simulink model "Tarea1-Simulacion"  (R2021b)
settings: Solver=VariableStepAuto  StartTime=0.0  StopTime=10  RelTol=1e-3
values from neighbouring files (symbols this model uses):
  Kc = Ksc (1:2)    [Tarea1-Marco_Rodriguez.m]
  Kd = Ksd (1:2)    [Tarea1-Marco_Rodriguez.m]
undefined symbols (not defined in the file or in its folder): DiscIntNeverNeededParam
libraries: cstblocks x10
settings Model: Creator=mvrb9  LastModifiedBy=mvrb9

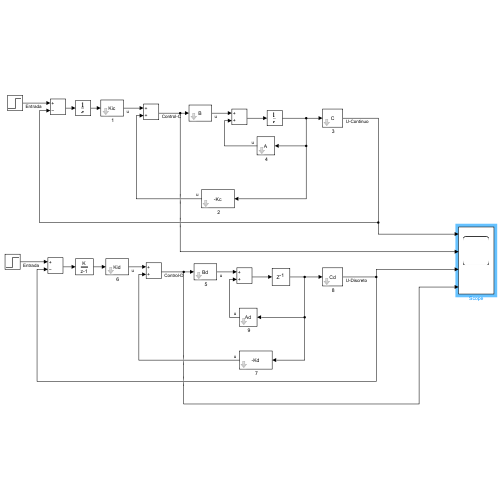
[thumbnail: Simulink's stored preview of the top-level diagram]
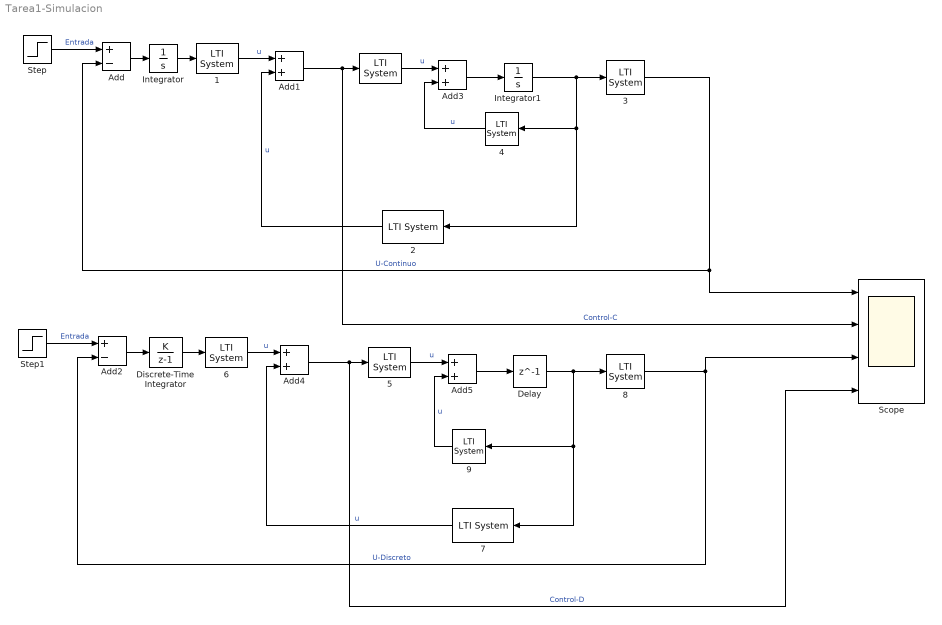
== system Tarea1-Simulacion ==
  " " : cstblocks/LTI System  sys=B  IC=[]
  " 1" : cstblocks/LTI System  sys=Kic  IC=[]
  " 2" : cstblocks/LTI System  sys=-Kc  IC=[]
  " 3" : cstblocks/LTI System  sys=C  IC=[]
  " 4" : cstblocks/LTI System  sys=A  IC=[]
  " 5" : cstblocks/LTI System  sys=Bd  IC=[]
  " 6" : cstblocks/LTI System  sys=Kid  IC=[]
  " 7" : cstblocks/LTI System  sys=-Kd  IC=[]
  " 8" : cstblocks/LTI System  sys=Cd  IC=[]
  " 9" : cstblocks/LTI System  sys=Ad  IC=[]
  Add : Sum  Inputs=+-
  Add{1,3..5} (4 alike) : Sum
  Add2 : Sum  Inputs=+-
  Delay : Delay  DelayLength=1  InitialCondition=0  SampleTime=0.01
  Discrete-Time Integrator : DiscreteIntegrator  IntegratorMethod=Accumulation: Forward Euler  SampleTime=0.01  ICPrevOutput=DiscIntNeverNeededParam  ICPrevScaledInput=DiscIntNeverNeededParam
  Integrator : Integrator
  Integrator1 : Integrator
  Scope : Scope  NumInputPorts=4
  Step : Step  SampleTime=0
  Step1 : Step  SampleTime=0
  wires:
  Step/1 -> Add/1  "Entrada"
  Add/1 -> Integrator/1
  Integrator/1 -> " 1"/1
  " 1"/1 -> Add1/1  "u"
  " "/1 -> Add3/1  "u"
  Add3/1 -> Integrator1/1
  " 3"/1 -> Scope/1, Add/2  "U-Continuo"
  " 4"/1 -> Add3/2  "u"
  Integrator1/1 -> " 2"/1, " 4"/1, " 3"/1
  " 2"/1 -> Add1/2  "u"
  Add1/1 -> Scope/2, " "/1  "Control-C"
  " 7"/1 -> Add4/2  "u"
  " 8"/1 -> Add2/2, Scope/3  "U-Discreto"
  Add2/1 -> Discrete-Time Integrator/1
  Discrete-Time Integrator/1 -> " 6"/1
  " 6"/1 -> Add4/1  "u"
  Add5/1 -> Delay/1
  Add4/1 -> Scope/4, " 5"/1  "Control-D"
  Step1/1 -> Add2/1  "Entrada"
  " 5"/1 -> Add5/1  "u"
  Delay/1 -> " 8"/1, " 7"/1, " 9"/1
  " 9"/1 -> Add5/2  "u"
